simulink model "quadcopter_model"  (R2024b)
settings: Solver=VariableStepAuto  StartTime=0.0  StopTime=10.0  RelTol=1e-3
undefined symbols (not defined in the file): g, Jx, Jy, Jz, k, l, m
libraries: simulink x4
settings Model: Creator=seecware  LastModifiedBy=seecware

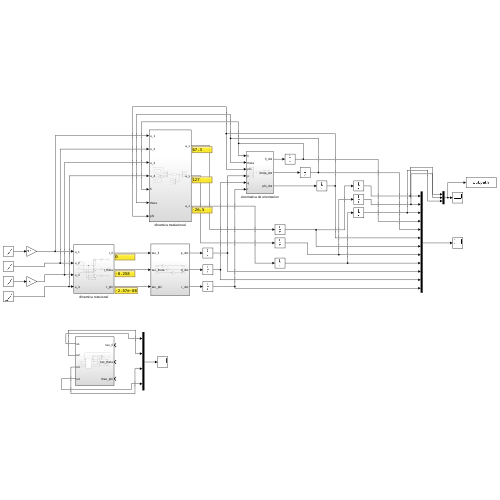
[thumbnail: Simulink's stored preview of the top-level diagram]
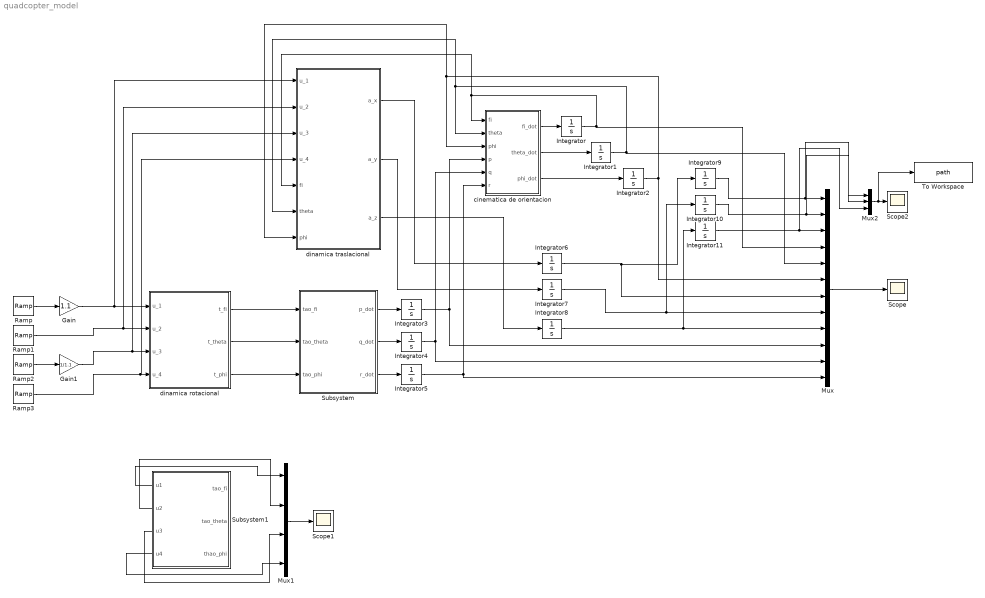
== system quadcopter_model ==
  Gain : Gain  Gain=1.1
  Gain1 : Gain  Gain=1/1.1
  Integrator{,1..11} (12 alike) : Integrator
  Mux : Mux  Inputs=12
  Mux1 : Mux
  Mux2 : Mux  Inputs=3
  Ramp{,1..3} (4 alike) : simulink/Sources/Ramp  slope=1  start=1  InitialOutput=0
  Scope : Scope
  Scope1 : Scope
  Scope2 : Scope
  Subsystem : Subsystem
  Subsystem1 : Subsystem
  To Workspace : ToWorkspace  VariableName=path  SaveFormat=Timeseries  SampleTime=-1
  cinematica de orientacion : Subsystem
  dinamica rotacional : Subsystem
  dinamica traslacional : Subsystem
  wires:
  cinematica de orientacion/1(fi_dot) -> Integrator/1
  cinematica de orientacion/2(theta_dot) -> Integrator1/1
  cinematica de orientacion/3(phi_dot) -> Integrator2/1
  Integrator/1 -> Mux/4, cinematica de orientacion/1(fi), dinamica traslacional/5(fi)
  Integrator1/1 -> Mux/5, cinematica de orientacion/2(theta), dinamica traslacional/6(theta)
  Integrator2/1 -> dinamica traslacional/7(phi), cinematica de orientacion/3(phi), Mux/6
  Subsystem/1(p_dot) -> Integrator3/1
  Subsystem/2(q_dot) -> Integrator4/1
  Subsystem/3(r_dot) -> Integrator5/1
  Integrator3/1 -> Mux/10, cinematica de orientacion/4(p)
  Integrator4/1 -> cinematica de orientacion/5(q), Mux/11
  Integrator5/1 -> cinematica de orientacion/6(r), Mux/12
  dinamica rotacional/1(t_fi) -> Subsystem/1(tao_fi)
  dinamica rotacional/2(t_theta) -> Subsystem/2(tao_theta)
  dinamica rotacional/3(t_phi) -> Subsystem/3(tao_phi)
  Integrator6/1 -> Integrator9/1, Mux/7
  Integrator7/1 -> Integrator10/1, Mux/8
  Integrator8/1 -> Integrator11/1, Mux/9
  dinamica traslacional/1(a_x) -> Integrator6/1
  dinamica traslacional/2(a_y) -> Integrator7/1
  dinamica traslacional/3(a_z) -> Integrator8/1
  Integrator9/1 -> Mux2/1, Mux/1
  Integrator10/1 -> Mux2/2, Mux/2
  Subsystem1/1(u1) -> Mux1/1
  Subsystem1/2(u2) -> Mux1/2
  Subsystem1/3(u3) -> Mux1/3
  Subsystem1/4(u4) -> Mux1/4
  Mux/1 -> Scope/1
  Integrator11/1 -> Mux2/3, Mux/3
  Mux1/1 -> Scope1/1
  Ramp/1 -> Gain/1
  Ramp1/1 -> dinamica traslacional/2(u_2), dinamica rotacional/2(u_2)
  Ramp2/1 -> Gain1/1
  Ramp3/1 -> dinamica traslacional/4(u_4), dinamica rotacional/4(u_4)
  Mux2/1 -> To Workspace/1, Scope2/1
  Gain/1 -> dinamica traslacional/1(u_1), dinamica rotacional/1(u_1)
  Gain1/1 -> dinamica traslacional/3(u_3), dinamica rotacional/3(u_3)

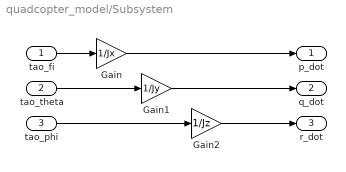
== system quadcopter_model/Subsystem ==
  tao_fi : Inport
  tao_theta : Inport  Port=2
  tao_phi : Inport  Port=3
  Gain : Gain  Gain=1/Jx
  Gain1 : Gain  Gain=1/Jy
  Gain2 : Gain  Gain=1/Jz
  p_dot : Outport
  q_dot : Outport  Port=2
  r_dot : Outport  Port=3
  wires:
  Gain/1 -> p_dot/1
  Gain2/1 -> r_dot/1
  tao_phi/1 -> Gain2/1
  tao_theta/1 -> Gain1/1
  tao_fi/1 -> Gain/1
  Gain1/1 -> q_dot/1

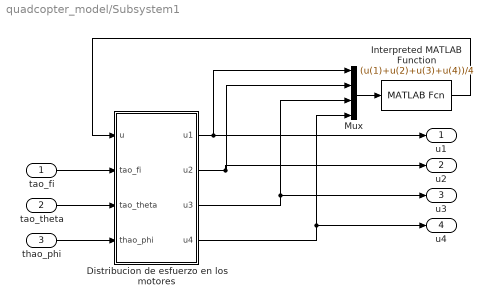
== system quadcopter_model/Subsystem1 ==
  tao_fi : Inport
  tao_theta : Inport  Port=2
  thao_phi : Inport  Port=3
  Distribucion de esfuerzo en los motores : Subsystem
  Interpreted MATLAB Function : MATLABFcn  MATLABFcn=(u(1)+u(2)+u(3)+u(4))/4
  Mux : Mux
  u1 : Outport
  u2 : Outport  Port=2
  u3 : Outport  Port=3
  u4 : Outport  Port=4
  wires:
  tao_theta/1 -> Distribucion de esfuerzo en los motores/3(tao_theta)
  Interpreted MATLAB Function/1 -> Distribucion de esfuerzo en los motores/1(u)
  thao_phi/1 -> Distribucion de esfuerzo en los motores/4(thao_phi)
  Distribucion de esfuerzo en los motores/1(u1) -> u1/1, Mux/1
  Distribucion de esfuerzo en los motores/2(u2) -> u2/1, Mux/2
  tao_fi/1 -> Distribucion de esfuerzo en los motores/2(tao_fi)
  Distribucion de esfuerzo en los motores/3(u3) -> u3/1, Mux/3
  Mux/1 -> Interpreted MATLAB Function/1
  Distribucion de esfuerzo en los motores/4(u4) -> u4/1, Mux/4

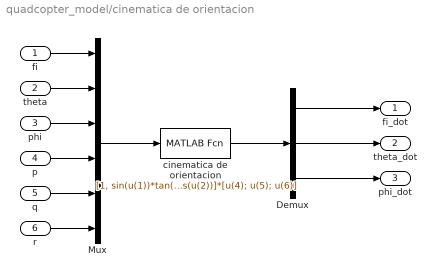
== system quadcopter_model/cinematica de orientacion ==
  fi : Inport
  theta : Inport  Port=2
  phi : Inport  Port=3
  p : Inport  Port=4
  q : Inport  Port=5
  r : Inport  Port=6
  Demux : Demux  Outputs=3
  Mux : Mux  Inputs=6
  cinematica de orientacion : MATLABFcn  MATLABFcn=[1, sin(u(1))*tan(u(2)), cos(u(1))*tan(u(2)); 0, cos(u(1)), -sin(u(1)); 0 sin(u(1))*cos(u(2)), cos(u(1))*cos(u(2))]*[u(4); u(5); u(6)]
  fi_dot : Outport
  theta_dot : Outport  Port=2
  phi_dot : Outport  Port=3
  wires:
  phi/1 -> Mux/3
  Demux/1 -> fi_dot/1
  cinematica de orientacion/1 -> Demux/1
  theta/1 -> Mux/2
  r/1 -> Mux/6
  p/1 -> Mux/4
  Demux/2 -> theta_dot/1
  Mux/1 -> cinematica de orientacion/1
  Demux/3 -> phi_dot/1
  q/1 -> Mux/5
  fi/1 -> Mux/1

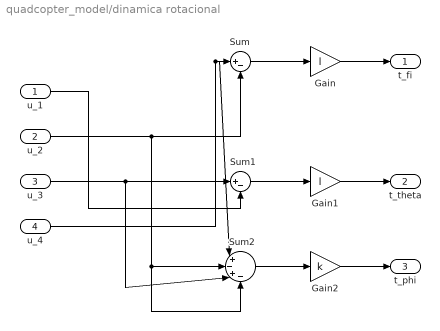
== system quadcopter_model/dinamica rotacional ==
  u_1 : Inport
  u_2 : Inport  Port=2
  u_3 : Inport  Port=3
  u_4 : Inport  Port=4
  Gain : Gain  Gain=l
  Gain1 : Gain  Gain=l
  Gain2 : Gain  Gain=k
  Sum : Sum  Inputs=|+-
  Sum1 : Sum  Inputs=|+-
  Sum2 : Sum  Inputs=|+-+-
  t_fi : Outport
  t_theta : Outport  Port=2
  t_phi : Outport  Port=3
  wires:
  Gain2/1 -> t_phi/1
  Gain/1 -> t_fi/1
  Gain1/1 -> t_theta/1
  u_4/1 -> Sum2/1, Sum/1
  u_3/1 -> Sum2/3, Sum1/1
  Sum2/1 -> Gain2/1
  u_1/1 -> Sum1/2
  Sum/1 -> Gain/1
  u_2/1 -> Sum2/4, Sum2/2, Sum/2
  Sum1/1 -> Gain1/1

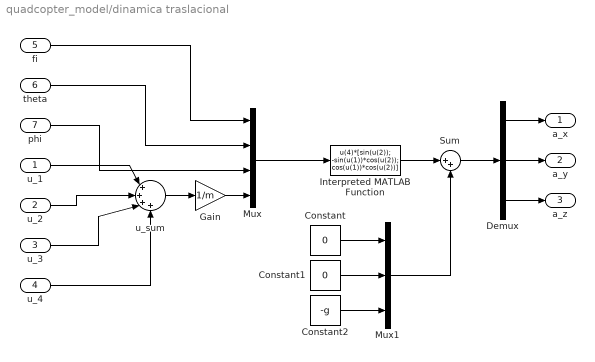
== system quadcopter_model/dinamica traslacional ==
  u_1 : Inport
  u_2 : Inport  Port=2
  u_3 : Inport  Port=3
  u_4 : Inport  Port=4
  fi : Inport  Port=5
  theta : Inport  Port=6
  phi : Inport  Port=7
  Constant : Constant  Value=0
  Constant1 : Constant  Value=0
  Constant2 : Constant  Value=-g
  Demux : Demux  Outputs=3
  Gain : Gain  Gain=1/m
  Interpreted MATLAB Function : MATLABFcn  MATLABFcn=u(4)*[sin(u(2)); -sin(u(1))*cos(u(2)); cos(u(1))*cos(u(2))]
  Mux : Mux
  Mux1 : Mux  Inputs=3
  Sum : Sum  Inputs=|++
  u_sum : Sum  Inputs=|++++
  a_x : Outport
  a_y : Outport  Port=2
  a_z : Outport  Port=3
  wires:
  u_sum/1 -> Gain/1
  u_4/1 -> u_sum/4
  fi/1 -> Mux/1
  u_1/1 -> u_sum/1
  phi/1 -> Mux/3
  u_3/1 -> u_sum/3
  Constant/1 -> Mux1/1
  theta/1 -> Mux/2
  Constant2/1 -> Mux1/3
  Constant1/1 -> Mux1/2
  Demux/3 -> a_z/1
  Mux/1 -> Interpreted MATLAB Function/1
  Demux/2 -> a_y/1
  Interpreted MATLAB Function/1 -> Sum/1
  Mux1/1 -> Sum/2
  Sum/1 -> Demux/1
  Gain/1 -> Mux/4
  u_2/1 -> u_sum/2
  Demux/1 -> a_x/1

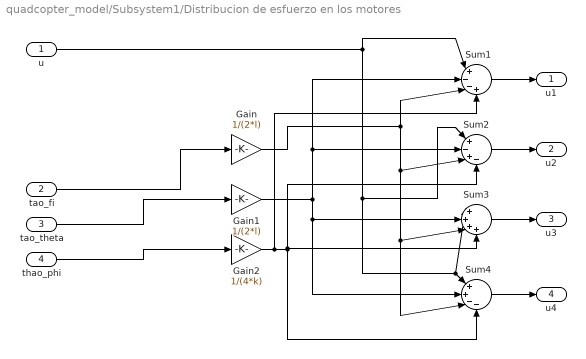
== system quadcopter_model/Subsystem1/Distribucion de esfuerzo en los motores ==
  u : Inport
  tao_fi : Inport  Port=2
  tao_theta : Inport  Port=3
  thao_phi : Inport  Port=4
  Gain : Gain  Gain=1/(2*l)
  Gain1 : Gain  Gain=1/(2*l)
  Gain2 : Gain  Gain=1/(4*k)
  Sum1 : Sum  Inputs=|+--+
  Sum2 : Sum  Inputs=|+-+-
  Sum3 : Sum  Inputs=|++++
  Sum4 : Sum  Inputs=|++--
  u1 : Outport
  u2 : Outport  Port=2
  u3 : Outport  Port=3
  u4 : Outport  Port=4
  wires:
  Gain2/1 -> Sum3/4, Sum2/4, Sum4/4, Sum1/4
  Gain1/1 -> Sum4/2, Sum3/2, Sum2/2, Sum1/2
  Sum3/1 -> u3/1
  thao_phi/1 -> Gain2/1
  tao_fi/1 -> Gain/1
  Sum4/1 -> u4/1
  Sum2/1 -> u2/1
  Sum1/1 -> u1/1
  Gain/1 -> Sum4/3, Sum3/3, Sum2/3, Sum1/3
  tao_theta/1 -> Gain1/1
  u/1 -> Sum2/1, Sum4/1, Sum3/1, Sum1/1
